simulink model "s2"  (Simulink 2.00)
settings: Solver=ode15s  StartTime=0.0  StopTime=tstop  MaxStep=0.0010  RelTol=1e-5  AbsTol=1e-5
values from neighbouring files (symbols this model uses):
  atten = exp(-(R/2)*sqrt(C/L)*d)    [M2.M]
  buffer_size = 20000    [M2.M]
  Epk = Vrated*sqrt(2/3)    [M2.M]
  LL = imag(ZL)/we    [M2.M]
  Ls = 0.1    [M2.M]
  Rc = 1000    [M2.M]
  RL = real(ZL)    [M2.M]
  Ro = 1000    [M2.M]
  tc = 1/60    (= 0.0166666666667)    [M2.M]
  tdelay = d*sqrt(L*C)    [M2.M]
  to = 1/60    (= 0.0166666666667)    [M2.M]
  we = 2*pi*60    (= 376.991118431)    [M1.M]    (also in M2.M)
  Zc = sqrt((r + j*we*l)/(j*we*c))    [M1.M]    (also in M2.M = sqrt(L/C))
settings Model: SaveTime=off  SaveOutput=off  ConsistencyChecking=off

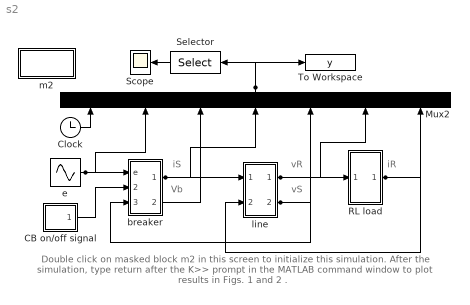
== system s2 ==
  note: iR
  note: Vb
  note: iS
  note: vS
  note: vR
  note: Double click on masked block m2 in this screen to initialize this simulation.
      | After the simulation, type return after the K>> prompt in the
      | MATLAB  command window to plot results in Figs. 1 and 2 .
  CB on/off signal : Subsystem  mask(Repeating table){@1=[0 10*Te 10*Te 1.1*tstop ], @2=[1 1 0 0  ]}
      mask prompts: @1 "Time values:"; @2 "Output values:"
      mask help:
      | Repeating table.
      | Enter values of time and output for first cycle.
      mask init:
      | period = max(@1); t = @1; y = @2;
      mask Help: Repeats cycle given in table. Time values should be monotonically increasing.
      mask Display: plot([t,t+period,t+2*period],[y,y,y])
  Clock : Clock
      settings: DeleteFcn=simclock BlockIsBeingDestroyed  PostSaveFcn=simclock Save
  m2 : Subsystem
      settings: OpenFcn=m2
      mask Type: Masked block of m2.m
      mask Help: Uses m2.m to initialize and plot
      mask Display: disp('Initialize\nand plot')
  Mux2 : Mux  Orientation=up  Inputs=7
  RL load : Subsystem
  Scope : Scope
      settings: TickLabels=on  TimeRange=0.25  YMin=-750000  YMax=750000  SaveToWorkspace=off  SaveName=ScopeData  LimitMaxRows=off  MaxRows=12000
  Selector : Selector  Orientation=left  Elements=[2 3 4 5 6 7]  InputPortWidth=7
  To Workspace : ToWorkspace  VariableName=y  SampleTime=0
      settings: Buffer=25000  Decimation=2
  breaker : Subsystem
  e : Sin  Amplitude=Epk  Frequency=we  Phase=pi/2  SampleTime=-1
  line : Subsystem
  wires:
  Mux2/1 -> Selector/1, To Workspace/1
  Selector/1 -> Scope/1
  Clock/1 -> Mux2/1
  CB on/off signal/1(out_1) -> breaker/2(CB on/off signal)
  e/1 -> breaker/1(e), Mux2/2
  breaker/2(vb) -> Mux2/3
  breaker/1(iS) -> line/1(iS), Mux2/4
  line/2(VS) -> breaker/3(vS), Mux2/5
  line/1("VR ") -> RL load/1(vR), Mux2/6
  RL load/1(iR) -> line/2(iR), Mux2/7

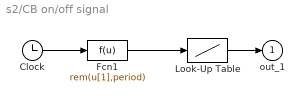
== system s2/CB on/off signal ==
  Clock : Clock
      settings: DeleteFcn=simclock BlockIsBeingDestroyed  PostSaveFcn=simclock Save
  Fcn1 : Fcn  Expr=rem(u[1],period)
  Look-Up Table : Lookup  InputValues=t  OutputValues=y
  out_1 : Outport  Port=1  InitialOutput=0
  wires:
  Look-Up Table/1 -> out_1/1
  Clock/1 -> Fcn1/1
  Fcn1/1 -> Look-Up Table/1

== system s2/m2 ==
  note: Masked block of m2.m to initalize s2.m
      | and plot results

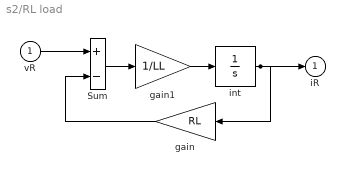
== system s2/RL load ==
  vR : Inport  Port=1  PortWidth=-1  SampleTime=-1
  Sum : Sum  Inputs=+-
  gain : Gain  Orientation=left  Gain=RL
  gain1 : Gain  Gain=1/LL
  int : Integrator  ExternalReset=none  InitialConditionSource=internal  InitialCondition=0  LimitOutput=off  UpperSaturationLimit=inf  LowerSaturationLimit=-inf  ShowSaturationPort=off  ShowStatePort=off  AbsoluteTolerance=auto
  iR : Outport  Port=1  InitialOutput=0
  wires:
  gain/1 -> Sum/2
  int/1 -> gain/1, iR/1
  vR/1 -> Sum/1
  Sum/1 -> gain1/1
  gain1/1 -> int/1

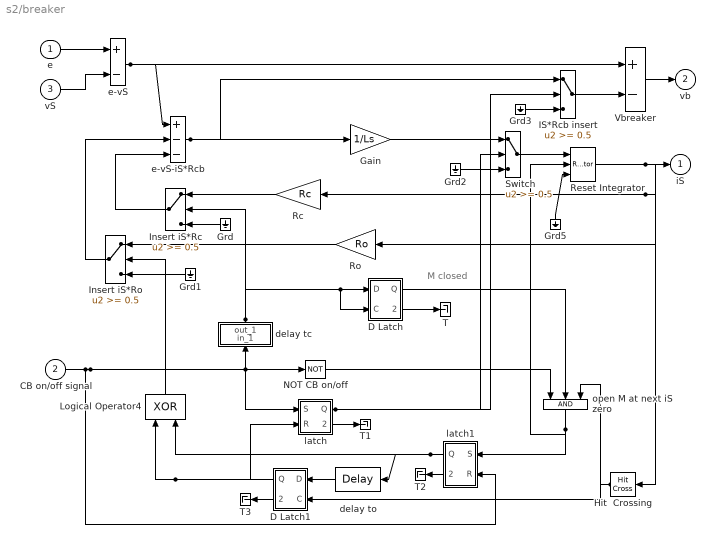
== system s2/breaker ==
  note: M closed
  e : Inport  Port=1  PortWidth=-1  SampleTime=-1
  CB on/off signal : Inport  Port=2  PortWidth=-1  SampleTime=-1
  vS : Inport  Port=3  PortWidth=-1  SampleTime=-1
  D Latch : Subsystem
  D Latch1 : Subsystem  Orientation=left
  Gain : Gain  Gain=1/Ls
  Grd : Ground  Orientation=left
  Grd1 : Ground  Orientation=left
  Grd2 : Ground
  Grd3 : Ground
  Grd5 : Ground  Orientation=up
  Hit  Crossing : HitCross  Orientation=left  HitCrossingOffset=1e-12  HitCrossingDirection=either  ShowOutputPort=on
  IS*Rcb insert : Switch  Threshold=0.5
  Insert iS*Rc : Switch  Orientation=left  Threshold=0.5
  Insert iS*Ro : Switch  Orientation=left  Threshold=0.5
  Logical Operator4 : Logic  Orientation=up  Operator=XOR  Inputs=2
  NOT CB on/off : Logic  Operator=NOT  Inputs=1
  Rc : Gain  Orientation=left  Gain=Rc
  Reset Integrator : ResetIntegrator  InitialCondition=0
  Ro : Gain  Orientation=left  Gain=Ro
  Switch : Switch  Threshold=0.5
  T{,1..3} (4 alike) : Terminator
  Vbreaker : Sum  Inputs=+-
  delay tc : Subsystem  Orientation=up
  delay to : TransportDelay  Orientation=left  DelayTime=to  InitialInput=0  BufferSize=20000
  e-vS : Sum  Inputs=+-
  e-vS-iS*Rcb : Sum  Inputs=+--
  latch : Subsystem
  latch1 : Subsystem  Orientation=left
  open M at next iS zero : Logic  Orientation=down  Operator=AND  Inputs=3
  iS : Outport  Port=1  InitialOutput=0
  vb : Outport  Port=2  InitialOutput=0
  wires:
  latch/1(Q) -> IS*Rcb insert/2, Switch/2
  latch/2(!Q) -> T1/1
  Ro/1 -> Insert iS*Ro/1
  e-vS-iS*Rcb/1 -> IS*Rcb insert/1, Gain/1
  Gain/1 -> Switch/1
  Rc/1 -> Insert iS*Rc/1
  Insert iS*Ro/1 -> e-vS-iS*Rcb/2
  Insert iS*Rc/1 -> e-vS-iS*Rcb/3
  CB on/off signal/1 -> NOT CB on/off/1, delay tc/1(in_1), latch/1(S), latch1/2(R)
  delay tc/1(out_1) -> D Latch/2(C), D Latch/1(D), Insert iS*Rc/2
  Logical Operator4/1 -> Insert iS*Ro/2
  Grd2/1 -> Switch/3
  Grd/1 -> Insert iS*Rc/3
  Grd1/1 -> Insert iS*Ro/3
  D Latch/2(!Q) -> T/1
  delay to/1 -> D Latch1/1(D)
  latch1/1(Q) -> Logical Operator4/2, delay to/1
  latch1/2(!Q) -> T2/1
  Hit  Crossing/1 -> D Latch1/2(C), open M at next iS zero/3
  D Latch1/2(!Q) -> T3/1
  D Latch1/1(Q) -> Logical Operator4/1, latch/2(R)
  Switch/1 -> Reset Integrator/1
  Reset Integrator/1 -> iS/1, Rc/1, Ro/1, Hit  Crossing/1
  Grd5/1 -> Reset Integrator/3
  D Latch/1(Q) -> open M at next iS zero/2
  NOT CB on/off/1 -> open M at next iS zero/1
  open M at next iS zero/1 -> latch1/1(S), Reset Integrator/2
  Vbreaker/1 -> vb/1
  e/1 -> e-vS/1
  IS*Rcb insert/1 -> Vbreaker/2
  e-vS/1 -> Vbreaker/1, e-vS-iS*Rcb/1
  vS/1 -> e-vS/2
  Grd3/1 -> IS*Rcb insert/3

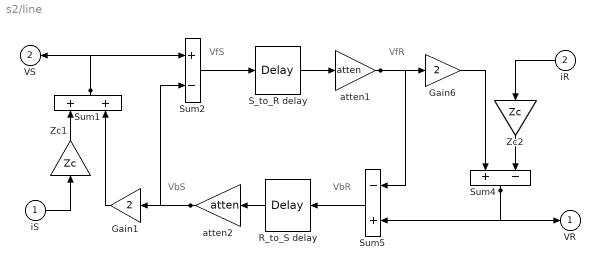
== system s2/line ==
  note: VbS
  note: VfS
  note: VbR
  note: VfR
  iS : Inport  Port=1  PortWidth=-1  SampleTime=-1
  iR : Inport  Orientation=left  Port=2  PortWidth=-1  SampleTime=-1
  Gain1 : Gain  Orientation=left  Gain=2
  Gain6 : Gain  Gain=2
  R_to_S delay : TransportDelay  Orientation=left  DelayTime=tdelay  InitialInput=0  BufferSize=buffer_size
  S_to_R delay : TransportDelay  DelayTime=tdelay  InitialInput=0  BufferSize=buffer_size
  Sum1 : Sum  Orientation=up  Inputs=++
  Sum2 : Sum  Inputs=+-
  Sum4 : Sum  Orientation=down  Inputs=+-
  Sum5 : Sum  Orientation=left  Inputs=-+
  Zc1 : Gain  Orientation=up  Gain=Zc
  Zc2 : Gain  Orientation=down  Gain=Zc
  atten1 : Gain  Gain=atten
  atten2 : Gain  Orientation=left  Gain=atten
  "VR " : Outport  Port=1  InitialOutput=0
  VS : Outport  Orientation=left  Port=2  InitialOutput=0
  wires:
  atten2/1 -> Sum2/2, Gain1/1
  R_to_S delay/1 -> atten2/1
  S_to_R delay/1 -> atten1/1
  Gain1/1 -> Sum1/2
  Gain6/1 -> Sum4/1
  Zc1/1 -> Sum1/1
  Sum2/1 -> S_to_R delay/1
  Zc2/1 -> Sum4/2
  Sum5/1 -> R_to_S delay/1
  Sum4/1 -> Sum5/2, "VR "/1
  iS/1 -> Zc1/1
  iR/1 -> Zc2/1
  Sum1/1 -> VS/1, Sum2/1
  atten1/1 -> Gain6/1, Sum5/1

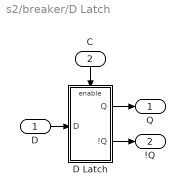
== system s2/breaker/D Latch ==
  D : Inport  Port=1  PortWidth=-1  SampleTime=-1
  C : Inport  Orientation=down  Port=2  PortWidth=-1  SampleTime=-1
  D Latch : Subsystem
  Q : Outport  Port=1  InitialOutput=0
  !Q : Outport  Port=2  InitialOutput=1
  wires:
  C/1 -> D Latch/Enable
  D Latch/1(Q) -> Q/1
  D/1 -> D Latch/1(D)
  D Latch/2(!Q) -> !Q/1

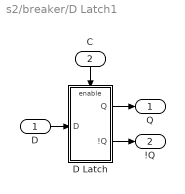
== system s2/breaker/D Latch1 ==
  D : Inport  Port=1  PortWidth=-1  SampleTime=-1
  C : Inport  Orientation=down  Port=2  PortWidth=-1  SampleTime=-1
  D Latch : Subsystem
  Q : Outport  Port=1  InitialOutput=0
  !Q : Outport  Port=2  InitialOutput=1
  wires:
  C/1 -> D Latch/Enable
  D Latch/1(Q) -> Q/1
  D/1 -> D Latch/1(D)
  D Latch/2(!Q) -> !Q/1

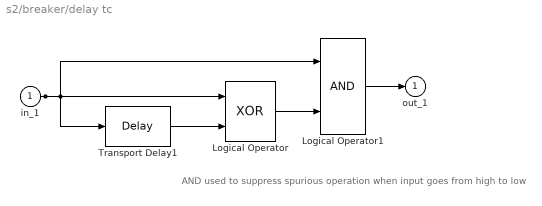
== system s2/breaker/delay tc ==
  note: AND  used to suppress
      | spurious operation when
      | input goes from high to low
  in_1 : Inport  Port=1  PortWidth=-1  SampleTime=-1
  Logical Operator : Logic  Operator=XOR  Inputs=2
  Logical Operator1 : Logic  Operator=AND  Inputs=2
  Transport Delay1 : TransportDelay  DelayTime=tc  InitialInput=0  BufferSize=20000
  out_1 : Outport  Port=1  InitialOutput=0
  wires:
  Transport Delay1/1 -> Logical Operator/2
  in_1/1 -> Logical Operator/1, Transport Delay1/1, Logical Operator1/1
  Logical Operator1/1 -> out_1/1
  Logical Operator/1 -> Logical Operator1/2

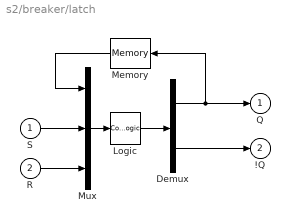
== system s2/breaker/latch ==
  S : Inport  Port=1  PortWidth=-1  SampleTime=-1
  R : Inport  Port=2  PortWidth=-1  SampleTime=-1
  Demux : Demux  Outputs=2
  Logic : CombinatorialLogic  TruthTable=[0 1;0 1;1 0;0 1;1 0;0 1;1 0;1 0]
  Memory : Memory  Orientation=left  X0=0  InheritSampleTime=on
  Mux : Mux  Inputs=3
  Q : Outport  Port=1  InitialOutput=0
  !Q : Outport  Port=2  InitialOutput=1
  wires:
  R/1 -> Mux/3
  S/1 -> Mux/2
  Memory/1 -> Mux/1
  Demux/1 -> Memory/1, Q/1
  Demux/2 -> !Q/1
  Logic/1 -> Demux/1
  Mux/1 -> Logic/1

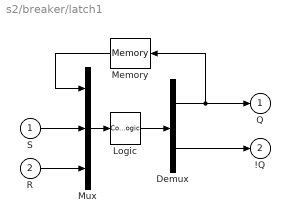
== system s2/breaker/latch1 ==
  S : Inport  Port=1  PortWidth=-1  SampleTime=-1
  R : Inport  Port=2  PortWidth=-1  SampleTime=-1
  Demux : Demux  Outputs=2
  Logic : CombinatorialLogic  TruthTable=[0 1;0 1;1 0;0 1;1 0;0 1;1 0;1 0]
  Memory : Memory  Orientation=left  X0=0  InheritSampleTime=on
  Mux : Mux  Inputs=3
  Q : Outport  Port=1  InitialOutput=0
  !Q : Outport  Port=2  InitialOutput=1
  wires:
  R/1 -> Mux/3
  S/1 -> Mux/2
  Memory/1 -> Mux/1
  Demux/1 -> Memory/1, Q/1
  Demux/2 -> !Q/1
  Logic/1 -> Demux/1
  Mux/1 -> Logic/1

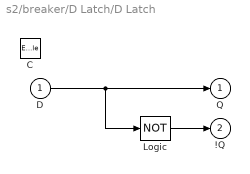
== system s2/breaker/D Latch/D Latch ==
  D : Inport  Port=1  PortWidth=-1  SampleTime=-1
  C : EnablePort
  Logic : Logic  Operator=NOT  Inputs=1
  Q : Outport  Port=1  InitialOutput=0
  !Q : Outport  Port=2  InitialOutput=1
  wires:
  Logic/1 -> !Q/1
  D/1 -> Q/1, Logic/1

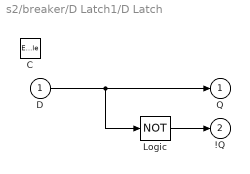
== system s2/breaker/D Latch1/D Latch ==
  D : Inport  Port=1  PortWidth=-1  SampleTime=-1
  C : EnablePort
  Logic : Logic  Operator=NOT  Inputs=1
  Q : Outport  Port=1  InitialOutput=0
  !Q : Outport  Port=2  InitialOutput=1
  wires:
  Logic/1 -> !Q/1
  D/1 -> Q/1, Logic/1
